simulink model "goertzel_algorithm5"  (R2021b)
settings: Solver=VariableStepAuto  StartTime=0.0  StopTime=20  FixedStep=0.001  RelTol=1e-3
values from neighbouring files (symbols this model uses):
  ac = 128    [create_simulink_model.m]
  coeff = 2*cos(omega)    [create_simulink_model.m]
  fcarrier = 10000    [create_simulink_model.m]
  fs = 1000000    [create_simulink_model.m]
  N = 1000    [create_simulink_model.m]
  omega = 2*pi*k/N    (= 0.0628318530718)    [create_simulink_model.m]
libraries: hdlsllib x2, simulink x1, commrandsrc3 x1
settings Model: Creator=caccolillo  LastModifiedBy=caccolillo

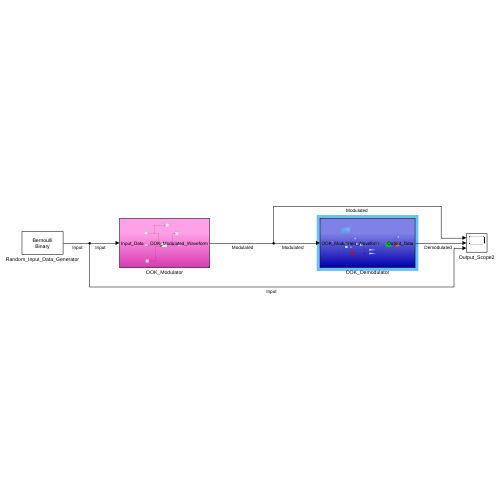
[thumbnail: Simulink's stored preview of the top-level diagram]
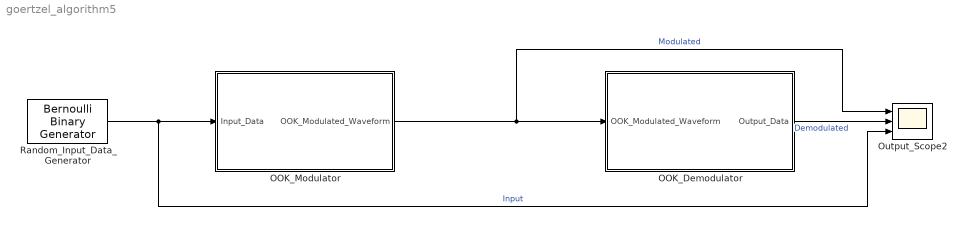
== system goertzel_algorithm5 ==
  OOK_Demodulator : Subsystem
  OOK_Modulator : Subsystem
  Output_Scope2 : Scope  NumInputPorts=3
  Random_Input_Data_Generator : commrandsrc3/Bernoulli Binary Generator  ProbabilityOfZero=0.5  SeedSource=Auto  Seed=0  SampleTime=1  SamplesPerFrame=1  OutputDataType=double  SimulateUsing=Interpreted execution
  wires:
  OOK_Modulator/1(OOK_Modulated_Waveform) -> OOK_Demodulator/1(OOK_Modulated_Waveform), Output_Scope2/1  "Modulated"
  OOK_Demodulator/1(Output_Data) -> Output_Scope2/2  "Demodulated"
  Random_Input_Data_Generator/1 -> Output_Scope2/3, OOK_Modulator/1(Input_Data)  "Input"

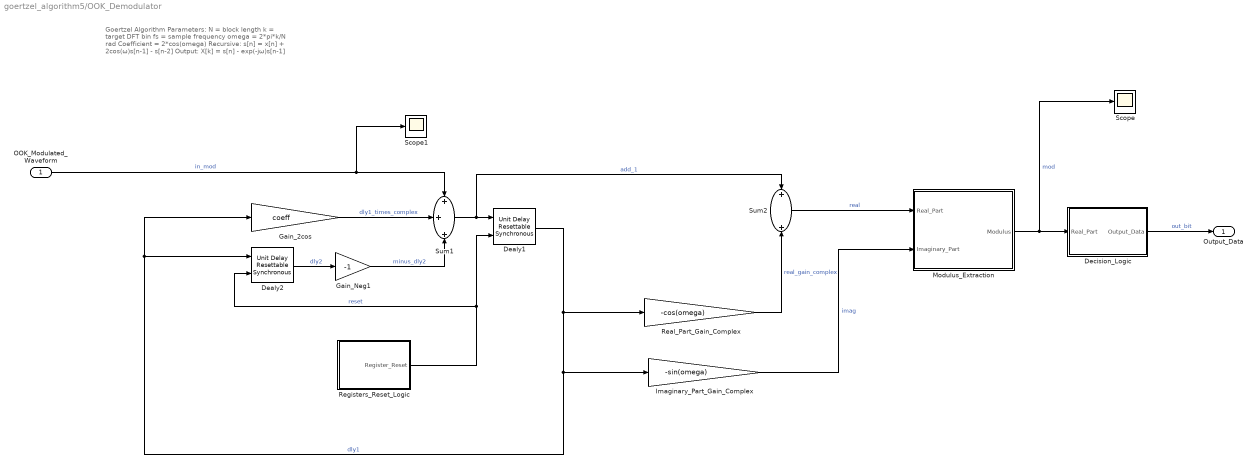
== system goertzel_algorithm5/OOK_Demodulator ==
  note: Goertzel Algorithm Parameters:
      | N = block length
      | k = target DFT bin
      | fs = sample frequency
      | omega = 2*pi*k/N rad
      | Coefficient = 2*cos(omega)
      |
      | Recursive: s[n] = x[n] + 2cos(ω)s[n-1] - s[n-2]
      | Output: X[k] = s[n] - exp(-jω)s[n-1]
  OOK_Modulated_Waveform : Inport
  Dealy1 : hdlsllib/Discrete/Unit Delay Resettable Synchronous  InitialCondition=0.0  SampleTime=-1
      settings: SourceProductBaseCode=SL
  Dealy2 : hdlsllib/Discrete/Unit Delay Resettable Synchronous  InitialCondition=0.0  SampleTime=-1
      settings: SourceProductBaseCode=SL
  Decision_Logic : Subsystem
  Gain_2cos : Gain  Gain=coeff
  Gain_Neg1 : Gain  Gain=-1
  Imaginary_Part_Gain_Complex : Gain  Gain=-sin(omega)
  Modulus_Extraction : Subsystem
  Real_Part_Gain_Complex : Gain  Gain=-cos(omega)
  Registers_Reset_Logic : Subsystem
  Scope : Scope
  Scope1 : Scope
  Sum1 : Sum  Inputs=+++
  Sum2 : Sum
  Output_Data : Outport
  wires:
  Gain_2cos/1 -> Sum1/2  "dly1_times_complex"
  Sum1/1 -> Dealy1/1, Sum2/1  "add_1"
  Decision_Logic/1(Output_Data) -> Output_Data/1  "out_bit"
  Dealy1/1 -> Real_Part_Gain_Complex/1, Imaginary_Part_Gain_Complex/1, Gain_2cos/1, Dealy2/1  "dly1"
  OOK_Modulated_Waveform/1 -> Scope1/1, Sum1/1  "in_mod"
  Registers_Reset_Logic/1(Register_Reset) -> Dealy1/2, Dealy2/2  "reset"
  Dealy2/1 -> Gain_Neg1/1  "dly2"
  Real_Part_Gain_Complex/1 -> Sum2/2  "real_gain_complex"
  Gain_Neg1/1 -> Sum1/3  "minus_dly2"
  Sum2/1 -> Modulus_Extraction/1(Real_Part)  "real"
  Imaginary_Part_Gain_Complex/1 -> Modulus_Extraction/2(Imaginary_Part)  "imag"
  Modulus_Extraction/1(Modulus) -> Scope/1, Decision_Logic/1(Real_Part)  "mod"

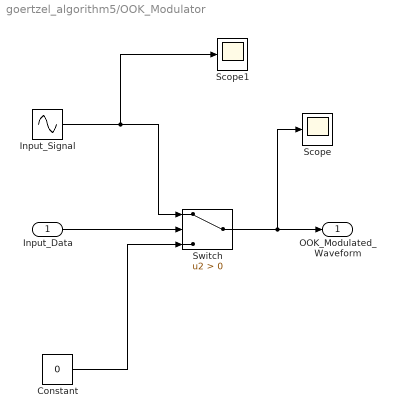
== system goertzel_algorithm5/OOK_Modulator ==
  Input_Data : Inport
  Constant : Constant  Value=0
  Input_Signal : Sin  Amplitude=ac  Frequency=2*pi*fcarrier  SampleTime=1/fs
  Scope : Scope
  Scope1 : Scope
  Switch : Switch  Criteria=u2 > Threshold
  OOK_Modulated_Waveform : Outport
  wires:
  Input_Data/1 -> Switch/2
  Input_Signal/1 -> Scope1/1, Switch/1
  Switch/1 -> Scope/1, OOK_Modulated_Waveform/1
  Constant/1 -> Switch/3

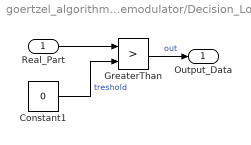
== system goertzel_algorithm5/OOK_Demodulator/Decision_Logic ==
  Real_Part : Inport
  Constant1 : Constant  Value=0
  GreaterThan : RelationalOperator  Operator=>  OutDataTypeStr=boolean  RndMeth=Simplest
  Output_Data : Outport
  wires:
  GreaterThan/1 -> Output_Data/1  "out"
  Real_Part/1 -> GreaterThan/1
  Constant1/1 -> GreaterThan/2  "treshold"

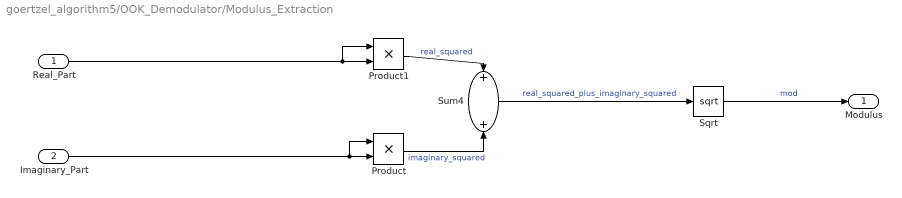
== system goertzel_algorithm5/OOK_Demodulator/Modulus_Extraction ==
  Real_Part : Inport
  Imaginary_Part : Inport  Port=2
  Product : Product
  Product1 : Product
  Sqrt : Sqrt  SaturateOnIntegerOverflow=on
  Sum4 : Sum
  Modulus : Outport
  wires:
  Sum4/1 -> Sqrt/1  "real_squared_plus_imaginary_squared"
  Product1/1 -> Sum4/1  "real_squared"
  Imaginary_Part/1 -> Product/1, Product/2
  Product/1 -> Sum4/2  "imaginary_squared"
  Sqrt/1 -> Modulus/1  "mod"
  Real_Part/1 -> Product1/1, Product1/2

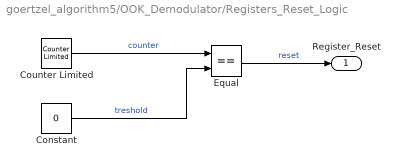
== system goertzel_algorithm5/OOK_Demodulator/Registers_Reset_Logic ==
  Constant : Constant  Value=0
  Counter Limited : simulink/Sources/Counter Limited  uplimit=N  tsamp=0.001
  Equal : RelationalOperator  Operator===  OutDataTypeStr=boolean  RndMeth=Simplest
  Register_Reset : Outport
  wires:
  Equal/1 -> Register_Reset/1  "reset"
  Counter Limited/1 -> Equal/1  "counter"
  Constant/1 -> Equal/2  "treshold"
